simulink model "RMS_computation"  (R2020a)
settings: Solver=FixedStepDiscrete  StartTime=0.0  StopTime=840000  RelTol=1e-3
libraries: hdlsllib x3, simulink x2
settings Model: FPTRunName=FPA_Reference  PacingRate=40  Creator=BuccelliLab  LastModifiedBy=diflo
settings SolverCC: AutoInsertRateTranBlk=on  MinimalZcImpactIntegration=on
settings DataIOCC: LimitDataPoints=on  SaveOutput=off  SaveTime=off  ReturnWorkspaceOutputs=off
settings OptimizationCC: BlockReduction=off  ConditionallyExecuteInputs=off  DefaultParameterBehavior=Inlined  LifeSpan=inf
settings DebuggingCC: SignalRangeChecking=warning  ReadBeforeWriteMsg=DisableAll  WriteAfterWriteMsg=DisableAll  WriteAfterReadMsg=DisableAll  AlgebraicLoopMsg=error  MultiTaskDSMMsg=none  SingleTaskRateTransMsg=error  ParameterDowncastMsg=warning  ParameterOverflowMsg=warning  AllowSymbolicDim=off  StrictBusMsg=ErrorOnBusTreatedAsVector  SFUnexpectedBacktrackingDiag=warning  SFNoUnconditionalDefaultTransitionDiag=warning  SFExecutionAtInitializationDiag=none  ArithmeticOperatorsInVariantConditions=warning
settings HardwareCC: ProdBitPerPointer=32  ProdBitPerSizeT=32  ProdBitPerPtrDiffT=32  ProdLargestAtomicFloat=None  ProdIntDivRoundTo=Undefined  ProdEndianess=Unspecified  ProdWordSize=32  ProdHWDeviceType=ASIC/FPGA->ASIC/FPGA  TargetBitPerPointer=64  TargetBitPerSizeT=64  TargetBitPerPtrDiffT=64  TargetLongLongMode=on  TargetIntDivRoundTo=Zero  TargetEndianess=LittleEndian  TargetWordSize=64  TargetHWDeviceType=Custom Processor->MATLAB Host Computer  ProdEqTarget=off
settings ModelReferenceCC: UpdateModelReferenceTargets=IfOutOfDate
settings SFSimCC: SFSimEcho=off  SimUseLocalCustomCode=off  CustomCodeUndefinedFunction=UseInterfaceOnly
settings RTWCC: RTWUseLocalCustomCode=off
settings CodeAppCC: StateflowObjectComments=on
settings GRTTargetCC: TargetLangStandard=C89/C90 (ANSI)
settings ConfigComp: CovScope=ReferencedModels  CovMetricSettings=dw  CovHtmlReporting=on  CovSaveCumulativeToWorkspaceVar=on  CovSaveSingleToWorkspaceVar=on  CovExternalEMLEnable=off  CovSFcnEnable=off

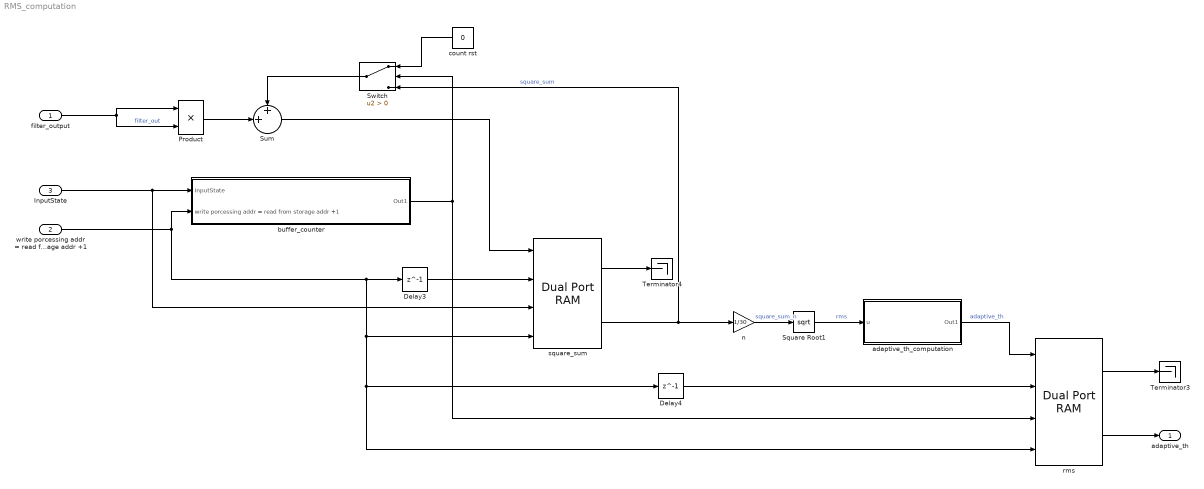
== system RMS_computation ==
  filter_output : Inport  OutDataTypeStr=uint16  PortDimensions=1  SampleTime=[1,0]
  write porcessing addr = read from storage addr +1 : Inport  Port=2  OutDataTypeStr=fixdt(0,9,0)  PortDimensions=1  SampleTime=[1,0]
  InputState : Inport  Port=3  OutDataTypeStr=boolean  PortDimensions=1  SampleTime=[1,0]
  Delay3 : Delay  DelayLength=1  InitialCondition=0
  Delay4 : Delay  DelayLength=1  InitialCondition=0
  Product : Product
  Square Root1 : Sqrt  OutDataTypeStr=uint16  SaturateOnIntegerOverflow=on
  Sum : Sum  Inputs=++|  OutDataTypeStr=uint64
  Switch : Switch  Criteria=u2 > Threshold  OutDataTypeStr=uint64
  Terminator3 : Terminator
  Terminator4 : Terminator
  adaptive_th_computation : Subsystem
  buffer_counter : Subsystem
  count rst : Constant  Value=0  OutDataTypeStr=uint64  SampleTime=-1
  n : Gain  Gain=1/30  OutDataTypeStr=fixdt(0,40,0)
  rms : hdlsllib/HDL RAMs/Dual Port RAM  ram_size=9
      settings: SourceProductBaseCode=SL
  square_sum : hdlsllib/HDL RAMs/Dual Port RAM  ram_size=9
      settings: SourceProductBaseCode=SL
  adaptive_th : Outport  OutDataTypeStr=uint16  PortDimensions=1  SampleTime=[1,0]
  wires:
  n/1 -> Square Root1/1  "square_sum_n"
  write porcessing addr = read from storage addr +1/1 -> Delay3/1, square_sum/4, Delay4/1, rms/4, buffer_counter/2(write porcessing addr = read from storage addr +1)
  count rst/1 -> Switch/1
  square_sum/2 -> Switch/3, n/1  "square_sum"
  Sum/1 -> square_sum/1
  buffer_counter/1(Out1) -> Switch/2, rms/3
  rms/1 -> Terminator3/1
  Product/1 -> Sum/2
  Delay4/1 -> rms/2
  Switch/1 -> Sum/1
  Delay3/1 -> square_sum/2
  square_sum/1 -> Terminator4/1
  InputState/1 -> buffer_counter/1(InputState), square_sum/3
  filter_output/1 -> Product/1, Product/2  "filter_out"
  rms/2 -> adaptive_th/1
  Square Root1/1 -> adaptive_th_computation/1(u)  "rms"
  adaptive_th_computation/1(Out1) -> rms/1  "adaptive_th"

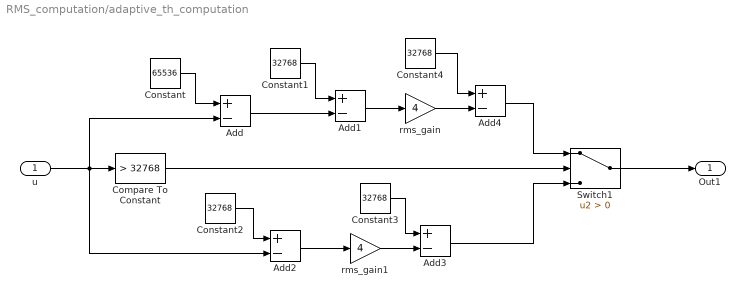
== system RMS_computation/adaptive_th_computation ==
  u : Inport
  Add{,1..4} (5 alike) : Sum  Inputs=+-  OutDataTypeStr=uint16
  Compare To Constant : simulink/Logic and Bit Operations/Compare To Constant  relop=>  const=32768  OutDataTypeStr=boolean
  Constant : Constant  Value=65536  OutDataTypeStr=uint16  SampleTime=-1
  Constant{1..4} (4 alike) : Constant  Value=32768  OutDataTypeStr=uint16  SampleTime=-1
  Switch1 : Switch  Criteria=u2 > Threshold
  rms_gain : Gain  Gain=4  OutDataTypeStr=uint16
  rms_gain1 : Gain  Gain=4  OutDataTypeStr=uint16
  Out1 : Outport
  wires:
  Switch1/1 -> Out1/1
  u/1 -> Compare To Constant/1, Add/2, Add2/2
  Add1/1 -> rms_gain/1
  Add2/1 -> rms_gain1/1
  Constant3/1 -> Add3/1
  rms_gain1/1 -> Add3/2
  Add4/1 -> Switch1/1
  Constant1/1 -> Add1/1
  rms_gain/1 -> Add4/2
  Constant4/1 -> Add4/1
  Add/1 -> Add1/2
  Compare To Constant/1 -> Switch1/2
  Constant/1 -> Add/1
  Constant2/1 -> Add2/1
  Add3/1 -> Switch1/3

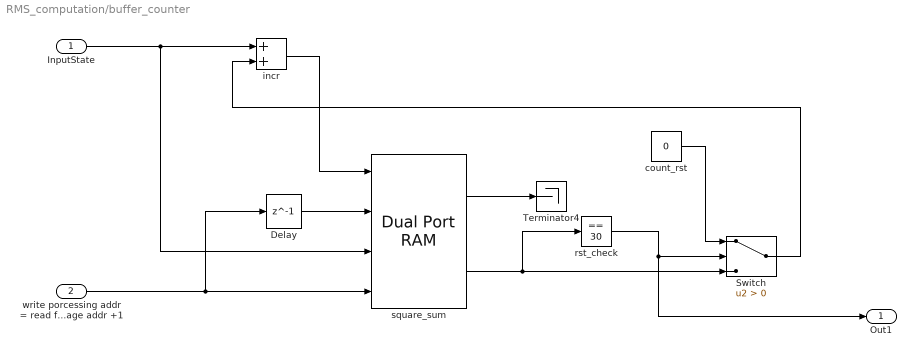
== system RMS_computation/buffer_counter ==
  InputState : Inport
  write porcessing addr = read from storage addr +1 : Inport  Port=2
  Delay : Delay  DelayLength=1  InitialCondition=0
  Switch : Switch  Criteria=u2 > Threshold  OutDataTypeStr=uint32
  Terminator4 : Terminator
  count_rst : Constant  Value=0  OutDataTypeStr=uint16  SampleTime=-1
  incr : Sum  AccumDataTypeStr=uint32
  rst_check : simulink/Logic and Bit Operations/Compare To Constant  relop===  const=30  OutDataTypeStr=boolean
  square_sum : hdlsllib/HDL RAMs/Dual Port RAM  ram_size=9
      settings: SourceProductBaseCode=SL
  Out1 : Outport
  wires:
  rst_check/1 -> Switch/2, Out1/1
  write porcessing addr = read from storage addr +1/1 -> Delay/1, square_sum/4
  Switch/1 -> incr/2
  InputState/1 -> square_sum/3, incr/1
  incr/1 -> square_sum/1
  Delay/1 -> square_sum/2
  count_rst/1 -> Switch/1
  square_sum/1 -> Terminator4/1
  square_sum/2 -> Switch/3, rst_check/1
